simulink library "csu_srp_solar_radiation_model_lib"  (R2014b)
settings: Solver=ode45  SolverMode=SingleTasking  StartTime=0.0  StopTime=10.0  RelTol=1e-3
values from neighbouring files (symbols this model uses):
  eph_pos_s2m_mcmf = eph_pos_m2s_mcmf .* -1    [csu_eph_spice_prep.m]
  eph_time_step_size = 1    [csu_eph_spice_init.m]
  ini_epoch_seconds = gbl_param.epoch_seconds    [csu_ini_initial_conditions_init.m]
undefined symbols (not defined in the file or in its folder): gbl_param, srp_K
libraries: util_common_lib x4, util_info_lib x2, util_quat_lib x2, csu_srp_solar_radiation_model_lib x2
settings Model: ExtModeAutoUpdateStatusClock=off  Creator=daniloviazzo  LastModifiedBy=mstewart

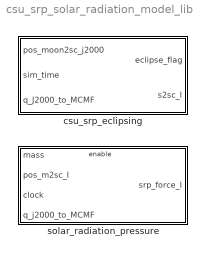
== system csu_srp_solar_radiation_model_lib ==
  csu_srp_eclipsing : Subsystem
  solar_radiation_pressure : Subsystem

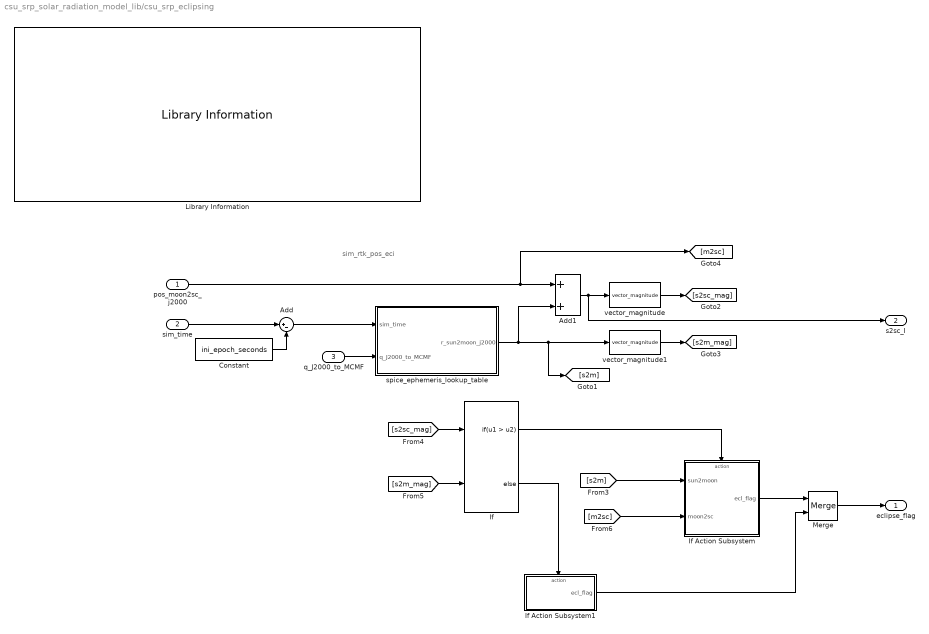
== system csu_srp_solar_radiation_model_lib/csu_srp_eclipsing ==
  note: sim_rtk_pos_eci
  pos_moon2sc_j2000 : Inport
  sim_time : Inport  Port=2
  q_J2000_to_MCMF : Inport  Port=3
  Add : Sum  Inputs=|+-
  Add1 : Sum
  Constant : Constant  Value=ini_epoch_seconds
  If : If  NumInputs=2  IfExpression=u1 > u2
  If Action Subsystem : Subsystem  TreatAsAtomicUnit=on
  If Action Subsystem1 : Subsystem  TreatAsAtomicUnit=on
  Library Information : util_info_lib/Library Information  owner='NONE'
  Merge : Merge
  spice_ephemeris_lookup_table : Subsystem
  vector_magnitude : util_common_lib/vector_magnitude  SystemSampleTime=-1
  vector_magnitude1 : util_common_lib/vector_magnitude  SystemSampleTime=-1
  eclipse_flag : Outport
  s2sc_I : Outport  Port=2
  wires:
  [m2sc] -> If Action Subsystem/2(moon2sc)
  [s2m_mag] -> If/2
  [s2sc_mag] -> If/1
  vector_magnitude1/1 -> [s2m_mag]
  vector_magnitude/1 -> [s2sc_mag]
  [s2m] -> If Action Subsystem/1(sun2moon)
  spice_ephemeris_lookup_table/1(r_sun2moon_j2000) -> [s2m], vector_magnitude1/1, Add1/2
  Add1/1 -> s2sc_I/1, vector_magnitude/1
  Merge/1 -> eclipse_flag/1
  If Action Subsystem/1(ecl_flag) -> Merge/1
  If Action Subsystem1/1(ecl_flag) -> Merge/2
  If/2 -> If Action Subsystem1/Action
  If/1 -> If Action Subsystem/Action
  pos_moon2sc_j2000/1 -> Add1/1, [m2sc]
  sim_time/1 -> Add/1
  Constant/1 -> Add/2
  Add/1 -> spice_ephemeris_lookup_table/1(sim_time)
  q_J2000_to_MCMF/1 -> spice_ephemeris_lookup_table/2(q_J2000_to_MCMF)

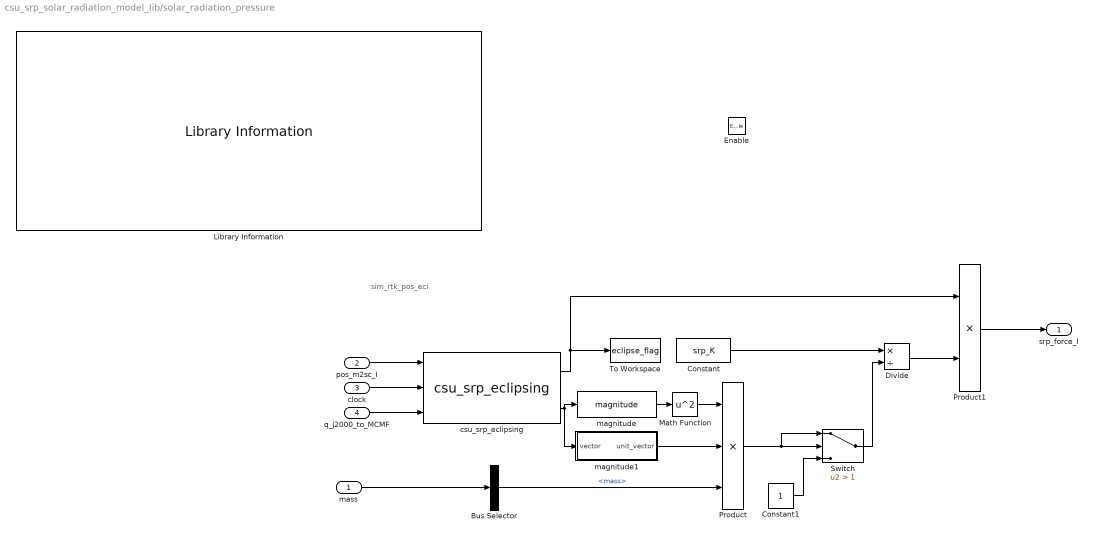
== system csu_srp_solar_radiation_model_lib/solar_radiation_pressure ==
  note: sim_rtk_pos_eci
  mass : Inport
  pos_m2sc_I : Inport  Port=2
  clock : Inport  Port=3
  q_j2000_to_MCMF : Inport  Port=4
  Enable : EnablePort
  Bus Selector : BusSelector  OutputSignals=mass
  Constant : Constant  Value=srp_K
  Constant1 : Constant
  Divide : Product  Inputs=*/
  Library Information : util_info_lib/Library Information  owner='NONE'
  Math Function : Math  Operator=square  SaturateOnIntegerOverflow=on
  Product : Product  Inputs=3
  Product1 : Product
  Switch : Switch  Criteria=u2 > Threshold  Threshold=1
  To Workspace : ToWorkspace  VariableName=eclipse_flag  SaveFormat=Timeseries  SampleTime=-1
  csu_srp_eclipsing : csu_srp_solar_radiation_model_lib/csu_srp_eclipsing
  magnitude : csu_srp_solar_radiation_model_lib/csu_srp_eclipsing/magnitude
  magnitude1 : Subsystem
  srp_force_I : Outport
  wires:
  Constant/1 -> Divide/1
  pos_m2sc_I/1 -> csu_srp_eclipsing/1
  clock/1 -> csu_srp_eclipsing/2
  q_j2000_to_MCMF/1 -> csu_srp_eclipsing/3
  csu_srp_eclipsing/1 -> Product1/1, To Workspace/1
  csu_srp_eclipsing/2 -> magnitude/1, magnitude1/1(vector)
  magnitude/1 -> Math Function/1
  mass/1 -> Bus Selector/1
  Product/1 -> Switch/1, Switch/2
  Switch/1 -> Divide/2
  Constant1/1 -> Switch/3
  Divide/1 -> Product1/2
  Product1/1 -> srp_force_I/1
  Math Function/1 -> Product/1
  magnitude1/1(unit_vector) -> Product/2
  Bus Selector/1 -> Product/3  "<mass>"

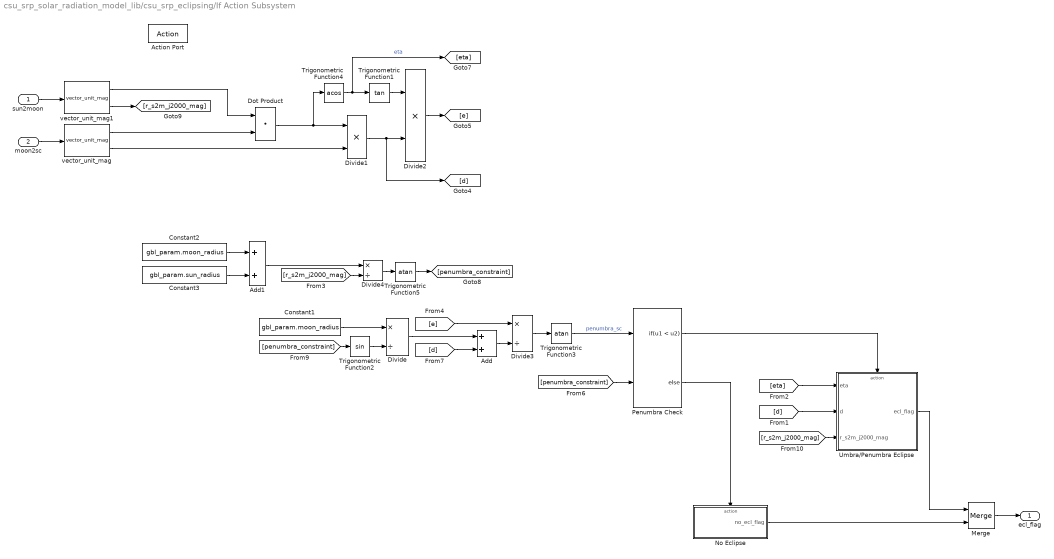
== system csu_srp_solar_radiation_model_lib/csu_srp_eclipsing/If Action Subsystem ==
  sun2moon : Inport
  moon2sc : Inport  Port=2
  Action Port : ActionPort
  Add : Sum
  Add1 : Sum
  Constant1 : Constant  Value=gbl_param.moon_radius
  Constant2 : Constant  Value=gbl_param.moon_radius
  Constant3 : Constant  Value=gbl_param.sun_radius
  Divide : Product  Inputs=*/
  Divide1 : Product  Inputs=**
  Divide2 : Product  Inputs=**
  Divide3 : Product  Inputs=*/
  Divide4 : Product  Inputs=*/
  Dot Product : DotProduct  InputSameDT=on  OutDataTypeStr=Inherit: Inherit via internal rule
  Merge : Merge
  No Eclipse : Subsystem  TreatAsAtomicUnit=on
  Penumbra Check : If  NumInputs=2  IfExpression=u1 < u2
  Trigonometric Function1 : Trigonometry  Operator=tan
  Trigonometric Function2 : Trigonometry
  Trigonometric Function3 : Trigonometry  Operator=atan
  Trigonometric Function4 : Trigonometry  Operator=acos
  Trigonometric Function5 : Trigonometry  Operator=atan
  Umbra/Penumbra Eclipse : Subsystem  TreatAsAtomicUnit=on
  vector_unit_mag : util_common_lib/vector_unit_mag  SystemSampleTime=-1
  vector_unit_mag1 : util_common_lib/vector_unit_mag  SystemSampleTime=-1
  ecl_flag : Outport
  wires:
  vector_unit_mag1/2 -> [r_s2m_j2000_mag]
  Trigonometric Function3/1 -> Penumbra Check/1  "penumbra_sc"
  Umbra/Penumbra Eclipse/1(ecl_flag) -> Merge/1
  Merge/1 -> ecl_flag/1
  No Eclipse/1(no_ecl_flag) -> Merge/2
  Penumbra Check/2 -> No Eclipse/Action
  Penumbra Check/1 -> Umbra/Penumbra Eclipse/Action
  [d] -> Umbra/Penumbra Eclipse/2(d)
  moon2sc/1 -> vector_unit_mag/1
  vector_unit_mag/2 -> Divide1/2
  vector_unit_mag1/1 -> Dot Product/1
  vector_unit_mag/1 -> Dot Product/2
  sun2moon/1 -> vector_unit_mag1/1
  Dot Product/1 -> Divide1/1, Trigonometric Function4/1
  Divide2/1 -> [e]
  Trigonometric Function1/1 -> Divide2/1
  [penumbra_constraint] -> Trigonometric Function2/1
  Constant1/1 -> Divide/1
  Trigonometric Function2/1 -> Divide/2
  [e] -> Divide3/1
  Divide1/1 -> [d], Divide2/2
  Divide/1 -> Add/1
  [d] -> Add/2
  Add/1 -> Divide3/2
  Divide3/1 -> Trigonometric Function3/1
  Trigonometric Function4/1 -> [eta], Trigonometric Function1/1  "eta"
  [eta] -> Umbra/Penumbra Eclipse/1(eta)
  [penumbra_constraint] -> Penumbra Check/2
  [r_s2m_j2000_mag] -> Umbra/Penumbra Eclipse/3("r_s2m_j2000_mag ")
  Constant2/1 -> Add1/1
  Constant3/1 -> Add1/2
  Add1/1 -> Divide4/1
  Divide4/1 -> Trigonometric Function5/1
  Trigonometric Function5/1 -> [penumbra_constraint]
  [r_s2m_j2000_mag] -> Divide4/2

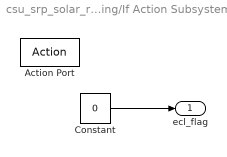
== system csu_srp_solar_radiation_model_lib/csu_srp_eclipsing/If Action Subsystem1 ==
  Action Port : ActionPort
  Constant : Constant  Value=0
  ecl_flag : Outport
  wires:
  Constant/1 -> ecl_flag/1

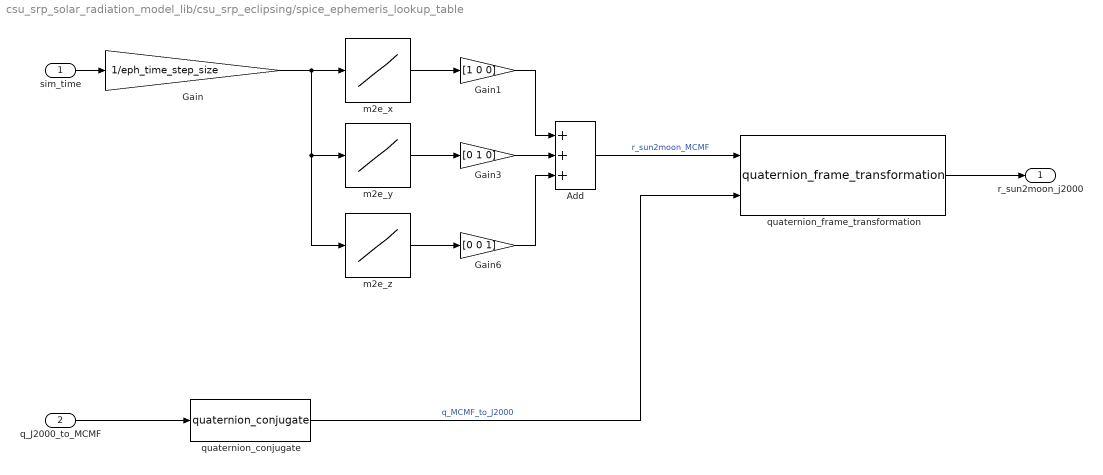
== system csu_srp_solar_radiation_model_lib/csu_srp_eclipsing/spice_ephemeris_lookup_table ==
  sim_time : Inport
  q_J2000_to_MCMF : Inport  Port=2
  Add : Sum  Inputs=+++
  Gain : Gain  Gain=1/eph_time_step_size
  Gain1 : Gain  Gain=[1 0 0]
  Gain3 : Gain  Gain=[0 1 0]
  Gain6 : Gain  Gain=[0 0 1]
  m2e_x : Lookup_n-D  NumberOfTableDimensions=1  BreakpointsForDimension1=[1:length(eph_pos_s2m_mcmf)]  Table=eph_pos_s2m_mcmf(:,1)  RndMeth=Simplest  InputSameDT=on
  m2e_y : Lookup_n-D  NumberOfTableDimensions=1  BreakpointsForDimension1=[1:length(eph_pos_s2m_mcmf)]  Table=eph_pos_s2m_mcmf(:,2)  RndMeth=Simplest  InputSameDT=on
  m2e_z : Lookup_n-D  NumberOfTableDimensions=1  BreakpointsForDimension1=[1:length(eph_pos_s2m_mcmf)]  Table=eph_pos_s2m_mcmf(:,3)  RndMeth=Simplest  InputSameDT=on
  quaternion_conjugate : util_quat_lib/quaternion_conjugate  SystemSampleTime=-1
  quaternion_frame_transformation : util_quat_lib/quaternion_frame_transformation  SystemSampleTime=-1
  r_sun2moon_j2000 : Outport
  wires:
  sim_time/1 -> Gain/1
  m2e_x/1 -> Gain1/1
  Gain/1 -> m2e_z/1, m2e_y/1, m2e_x/1
  m2e_y/1 -> Gain3/1
  m2e_z/1 -> Gain6/1
  Gain3/1 -> Add/2
  Gain1/1 -> Add/1
  Gain6/1 -> Add/3
  q_J2000_to_MCMF/1 -> quaternion_conjugate/1
  quaternion_frame_transformation/1 -> r_sun2moon_j2000/1
  quaternion_conjugate/1 -> quaternion_frame_transformation/2  "q_MCMF_to_J2000"
  Add/1 -> quaternion_frame_transformation/1  "r_sun2moon_MCMF"

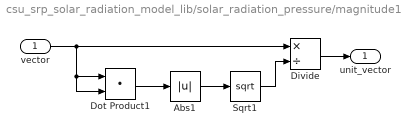
== system csu_srp_solar_radiation_model_lib/solar_radiation_pressure/magnitude1 ==
  vector : Inport
  Abs1 : Abs
  Divide : Product  Inputs=*/
  Dot Product1 : DotProduct  InputSameDT=on  OutDataTypeStr=Inherit: Inherit via internal rule
  Sqrt1 : Sqrt  SaturateOnIntegerOverflow=on
  unit_vector : Outport
  wires:
  Abs1/1 -> Sqrt1/1
  Sqrt1/1 -> Divide/2
  Dot Product1/1 -> Abs1/1
  vector/1 -> Dot Product1/2, Dot Product1/1, Divide/1
  Divide/1 -> unit_vector/1

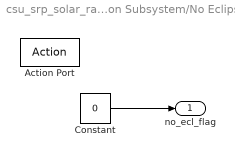
== system csu_srp_solar_radiation_model_lib/csu_srp_eclipsing/If Action Subsystem/No Eclipse ==
  Action Port : ActionPort
  Constant : Constant  Value=0
  no_ecl_flag : Outport
  wires:
  Constant/1 -> no_ecl_flag/1

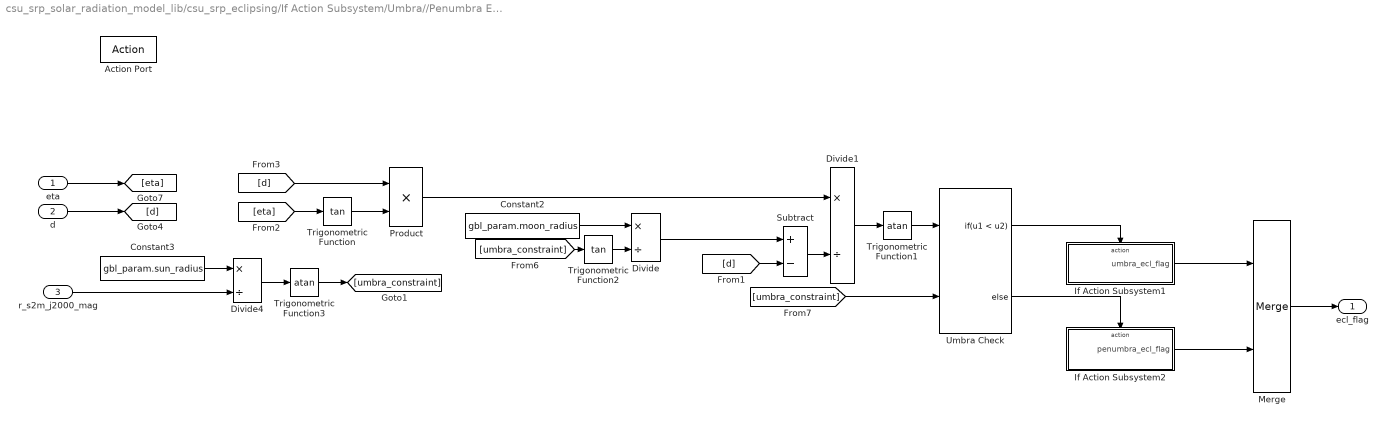
== system csu_srp_solar_radiation_model_lib/csu_srp_eclipsing/If Action Subsystem/Umbra//Penumbra Eclipse ==
  eta : Inport
  d : Inport  Port=2
  "r_s2m_j2000_mag " : Inport  Port=3
  Action Port : ActionPort
  Constant2 : Constant  Value=gbl_param.moon_radius
  Constant3 : Constant  Value=gbl_param.sun_radius
  Divide : Product  Inputs=*/
  Divide1 : Product  Inputs=*/
  Divide4 : Product  Inputs=*/
  If Action Subsystem1 : Subsystem  TreatAsAtomicUnit=on
  If Action Subsystem2 : Subsystem  TreatAsAtomicUnit=on
  Merge : Merge
  Product : Product
  Subtract : Sum  Inputs=+-
  Trigonometric Function : Trigonometry  Operator=tan
  Trigonometric Function1 : Trigonometry  Operator=atan
  Trigonometric Function2 : Trigonometry  Operator=tan
  Trigonometric Function3 : Trigonometry  Operator=atan
  Umbra Check : If  NumInputs=2  IfExpression=u1 < u2
  ecl_flag : Outport
  wires:
  Merge/1 -> ecl_flag/1
  If Action Subsystem2/1(penumbra_ecl_flag) -> Merge/2
  Umbra Check/2 -> If Action Subsystem2/Action
  If Action Subsystem1/1(umbra_ecl_flag) -> Merge/1
  Umbra Check/1 -> If Action Subsystem1/Action
  eta/1 -> [eta]
  d/1 -> [d]
  Constant2/1 -> Divide/1
  Divide/1 -> Subtract/1
  [d] -> Subtract/2
  [eta] -> Trigonometric Function/1
  [d] -> Product/1
  Trigonometric Function/1 -> Product/2
  Product/1 -> Divide1/1
  Subtract/1 -> Divide1/2
  Divide1/1 -> Trigonometric Function1/1
  Trigonometric Function1/1 -> Umbra Check/1
  [umbra_constraint] -> Trigonometric Function2/1
  [umbra_constraint] -> Umbra Check/2
  Trigonometric Function2/1 -> Divide/2
  Constant3/1 -> Divide4/1
  "r_s2m_j2000_mag "/1 -> Divide4/2
  Divide4/1 -> Trigonometric Function3/1
  Trigonometric Function3/1 -> [umbra_constraint]

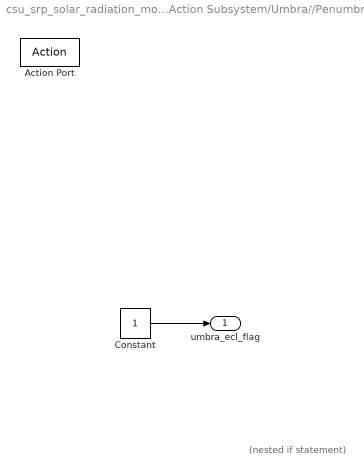
== system csu_srp_solar_radiation_model_lib/csu_srp_eclipsing/If Action Subsystem/Umbra//Penumbra Eclipse/If Action Subsystem1 ==
  note: (nested if statement)
  Action Port : ActionPort
  Constant : Constant
  umbra_ecl_flag : Outport
  wires:
  Constant/1 -> umbra_ecl_flag/1

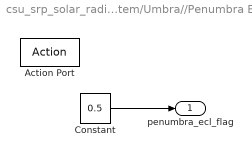
== system csu_srp_solar_radiation_model_lib/csu_srp_eclipsing/If Action Subsystem/Umbra//Penumbra Eclipse/If Action Subsystem2 ==
  Action Port : ActionPort
  Constant : Constant  Value=0.5
  penumbra_ecl_flag : Outport
  wires:
  Constant/1 -> penumbra_ecl_flag/1
